simulink model "cvicenie_2bm"  (R2024b)
settings: Solver=VariableStepAuto  StartTime=0.0  StopTime=2  RelTol=1e-3
values from neighbouring files (symbols this model uses):
  omega_0 = 2*pi/T    (= 3.14159265359)    [cvicenie_2b.m]
settings Model: Creator=Nergigante  LastModifiedBy=Nergigante

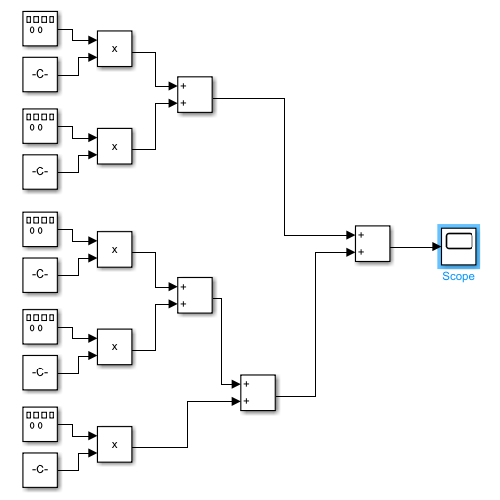
[thumbnail: Simulink's stored preview of the top-level diagram]
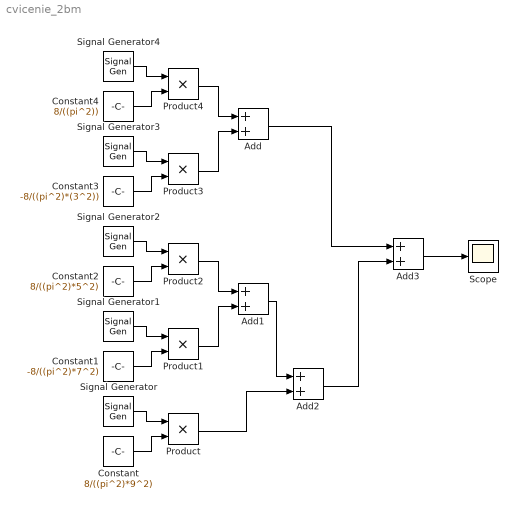
== system cvicenie_2bm ==
  Add{,1..3} (4 alike) : Sum
  Constant : Constant  Value=8/((pi^2)*9^2)
  Constant1 : Constant  Value=-8/((pi^2)*7^2)
  Constant2 : Constant  Value=8/((pi^2)*5^2)
  Constant3 : Constant  Value=-8/((pi^2)*(3^2))
  Constant4 : Constant  Value=8/((pi^2))
  Product{,1..4} (5 alike) : Product
  Scope : Scope
  Signal Generator : SignalGenerator  Frequency=9*omega_0  Units=rad/sec
  Signal Generator1 : SignalGenerator  Frequency=7*omega_0  Units=rad/sec
  Signal Generator2 : SignalGenerator  Frequency=5*omega_0  Units=rad/sec
  Signal Generator3 : SignalGenerator  Frequency=3*omega_0  Units=rad/sec
  Signal Generator4 : SignalGenerator  Frequency=omega_0  Units=rad/sec
  wires:
  Signal Generator/1 -> Product/1
  Constant/1 -> Product/2
  Constant1/1 -> Product1/2
  Signal Generator1/1 -> Product1/1
  Constant2/1 -> Product2/2
  Signal Generator2/1 -> Product2/1
  Constant3/1 -> Product3/2
  Signal Generator3/1 -> Product3/1
  Constant4/1 -> Product4/2
  Signal Generator4/1 -> Product4/1
  Product4/1 -> Add/1
  Product3/1 -> Add/2
  Product2/1 -> Add1/1
  Product1/1 -> Add1/2
  Add1/1 -> Add2/1
  Product/1 -> Add2/2
  Add/1 -> Add3/1
  Add2/1 -> Add3/2
  Add3/1 -> Scope/1
